simulink model "DWT"  (R2023a)
settings: Solver=ode45  StartTime=0.0  StopTime=4096+1024+100  RelTol=1e-3  EnableMultiTasking=on
PreLoadFcn:
  | xlrequire('imageData.mat'); xlrequire('PreLoadFcn');
PostLoadFcn:
  | open_system('DWT/Processor/Memory Controller','force'); pause(0.50); open_system('DWT');pause(0.50); close_system('DWT/Processor/Memory Controller');pause(0.50); close_system('DWT/Processor');
StopFcn:
  | xlrequire('StopFcn');
undefined symbols (not defined in the file): b1Init, b2Init
libraries: hdlBasic x212, dspindex x4, dspsnks4 x2, hdlUtilities x1, dspsrcs4 x1, vmcUtilities x1
(part 2 of 2)

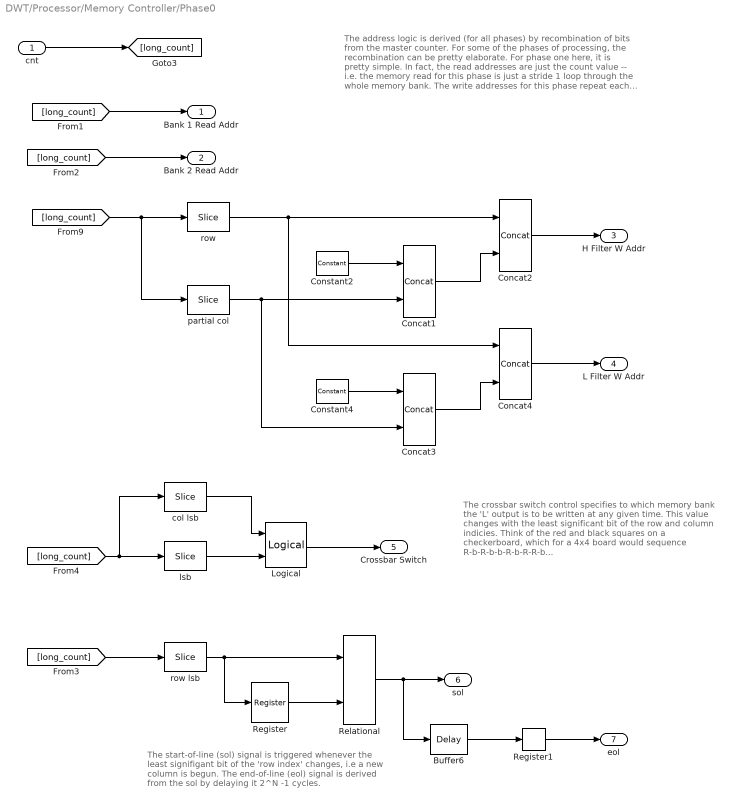
== system DWT/Processor/Memory Controller/Phase0 ==
  note: The address logic is derived (for all phases) by recombination
      | of bits from the master counter. For some of the phases of
      | processing, the recombination can be pretty elaborate.  For
      | phase one here, it is pretty simple.  In fact, the read addresses
      | are just the count value -- i.e. the memory read for this phase
      | is just a stride 1 loop through the whole memory bank.  The
      | write addresses for this phase repeat each address twice (data
      | is written to an address in one bank and then the same address
      | in the other bank for each filter).  The addresses increment by
      | one as each column is processed, and then jump to the next
      | column. A '1' is injected into the H address and a '0' into the 'L'
      | adress to write to the lower or upper half of memory, respectively.
  note: The crossbar switch control specifies to which memory
      | bank the 'L' output is to be written at any given time.
      | This value changes with the least significant bit of the
      | row and column indicies.  Think of the red and black
      | squares on a checkerboard, which for a 4x4 board would
      | sequence R-b-R-b-b-R-b-R-R-b...
  note: The start-of-line (sol) signal is triggered whenever the
      | least signifigant bit of the 'row index' changes, i.e a
      | new column is begun.  The end-of-line (eol) signal is
      | derived from the sol by delaying it 2^N -1 cycles.
  cnt : Inport
  Buffer6 : hdlBasic/Delay  rst=off  en=off  latency=power(2,N-1)-2  reg_retiming=off  XmcBlockStatus=1  maskContainerNames=group1  block_type=delay  block_config=sysgen:Delay_config
  Concat{1..4} (4 alike) : hdlBasic/Concat  num_inputs=2  XmcBlockStatus=1  maskContainerNames=group1  block_type=concat  block_config=sysgen:Concat_config
  Constant2 : hdlBasic/Constant  const=1  gui_display_data_type=Fixed-point  arith_type=Unsigned  n_bits=1  bin_pt=0  preci_type=Single  exp_width=8  frac_width=24  explicit_period=off  period=1  XmcBlockStatus=1  maskContainerNames=tabcontainer1  block_type=constant  block_config=sysgen:Constant_config
  Constant4 : hdlBasic/Constant  const=0  gui_display_data_type=Fixed-point  arith_type=Unsigned  n_bits=1  bin_pt=0  preci_type=Single  exp_width=8  frac_width=24  explicit_period=off  period=1  XmcBlockStatus=1  maskContainerNames=tabcontainer1  block_type=constant  block_config=sysgen:Constant_config
  Logical : hdlBasic/Logical  logical_function=XNOR  inputs=2  en=off  latency=0  precision=Full  arith_type=Unsigned  n_bits=8  bin_pt=2  align_bp=on  overflow=[]  quantization=[]  XmcBlockStatus=1  maskContainerNames=tabcontainer1  block_type=logical  block_config=sysgen:Logical_config
  Register : hdlBasic/Register  init=1  rst=off  en=off  XmcBlockStatus=1  maskContainerNames=tabcontainer1  block_type=register  block_config=sysgen:Register_config
  Register1 : hdlBasic/Register  init=0  rst=off  en=off  XmcBlockStatus=1  maskContainerNames=tabcontainer1  block_type=register  block_config=sysgen:Register_config
  Relational : hdlBasic/Relational  mode=a!=b  op_type=Bool  en=off  latency=0  XmcBlockStatus=1  maskContainerNames=tabcontainer1  block_type=relational  block_config=sysgen:Relational_config
  col lsb : hdlBasic/Slice  nbits=1  boolean_output=off  mode=Lower Bit Location + Width  bit1=0  base1=MSB of Input  bit0=M-1  base0=LSB of Input  XmcBlockStatus=1  maskContainerNames=group1  block_type=slice  block_config=sysgen:Slice_config
  lsb : hdlBasic/Slice  nbits=1  boolean_output=off  mode=Lower Bit Location + Width  bit1=0  base1=MSB of Input  bit0=0  base0=LSB of Input  XmcBlockStatus=1  maskContainerNames=group1  block_type=slice  block_config=sysgen:Slice_config
  partial col : hdlBasic/Slice  nbits=N-2  boolean_output=off  mode=Lower Bit Location + Width  bit1=0  base1=MSB of Input  bit0=1  base0=LSB of Input  XmcBlockStatus=1  maskContainerNames=group1  block_type=slice  block_config=sysgen:Slice_config
  row : hdlBasic/Slice  nbits=M  boolean_output=off  mode=Upper Bit Location + Width  bit1=0  base1=MSB of Input  bit0=N  base0=LSB of Input  XmcBlockStatus=1  maskContainerNames=group1  block_type=slice  block_config=sysgen:Slice_config
  row lsb : hdlBasic/Slice  nbits=1  boolean_output=off  mode=Lower Bit Location + Width  bit1=0  base1=MSB of Input  bit0=N-1  base0=LSB of Input  XmcBlockStatus=1  maskContainerNames=group1  block_type=slice  block_config=sysgen:Slice_config
  Bank 1 Read Addr : Outport  VectorParamsAs1DForOutWhenUnconnected=off
  Bank 2 Read Addr : Outport  Port=2  VectorParamsAs1DForOutWhenUnconnected=off
  H Filter W Addr : Outport  Port=3  VectorParamsAs1DForOutWhenUnconnected=off
  L Filter W Addr : Outport  Port=4  VectorParamsAs1DForOutWhenUnconnected=off
  Crossbar Switch : Outport  Port=5  VectorParamsAs1DForOutWhenUnconnected=off
  sol : Outport  Port=6  VectorParamsAs1DForOutWhenUnconnected=off
  eol : Outport  Port=7  VectorParamsAs1DForOutWhenUnconnected=off
  wires:
  [long_count] -> Bank 2 Read Addr/1
  [long_count] -> row lsb/1
  row lsb/1 -> Relational/1, Register/1
  Relational/1 -> sol/1, Buffer6/1
  Buffer6/1 -> Register1/1
  [long_count] -> lsb/1, col lsb/1
  Register/1 -> Relational/2
  [long_count] -> row/1, partial col/1
  row/1 -> Concat4/1, Concat2/1
  Constant2/1 -> Concat1/1
  Constant4/1 -> Concat3/1
  Concat3/1 -> Concat4/2
  partial col/1 -> Concat3/2, Concat1/2
  Concat1/1 -> Concat2/2
  [long_count] -> Bank 1 Read Addr/1
  Concat2/1 -> H Filter W Addr/1
  Concat4/1 -> L Filter W Addr/1
  Register1/1 -> eol/1
  cnt/1 -> [long_count]
  lsb/1 -> Logical/2
  col lsb/1 -> Logical/1
  Logical/1 -> Crossbar Switch/1

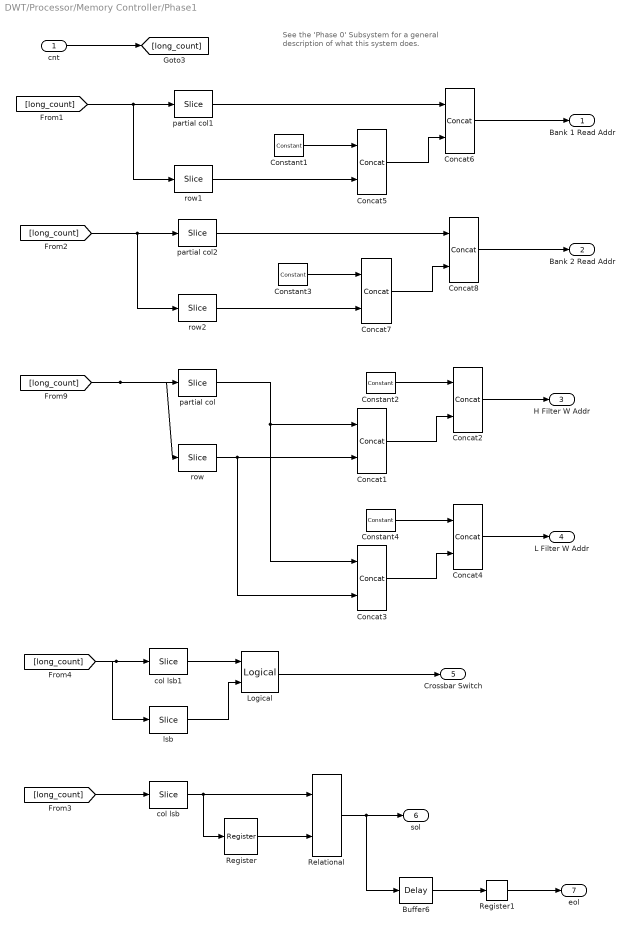
== system DWT/Processor/Memory Controller/Phase1 ==
  note: See the 'Phase 0' Subsystem for a general
      | description of what this system does.
  cnt : Inport
  Buffer6 : hdlBasic/Delay  rst=off  en=off  latency=power(2,N-1)-2  reg_retiming=off  XmcBlockStatus=1  maskContainerNames=group1  block_type=delay  block_config=sysgen:Delay_config
  Concat{1..8} (8 alike) : hdlBasic/Concat  num_inputs=2  XmcBlockStatus=1  maskContainerNames=group1  block_type=concat  block_config=sysgen:Concat_config
  Constant1 : hdlBasic/Constant  const=1  gui_display_data_type=Fixed-point  arith_type=Unsigned  n_bits=1  bin_pt=0  preci_type=Single  exp_width=8  frac_width=24  explicit_period=off  period=1  XmcBlockStatus=1  maskContainerNames=tabcontainer1  block_type=constant  block_config=sysgen:Constant_config
  Constant2 : hdlBasic/Constant  const=1  gui_display_data_type=Fixed-point  arith_type=Unsigned  n_bits=1  bin_pt=0  preci_type=Single  exp_width=8  frac_width=24  explicit_period=off  period=1  XmcBlockStatus=1  maskContainerNames=tabcontainer1  block_type=constant  block_config=sysgen:Constant_config
  Constant3 : hdlBasic/Constant  const=0  gui_display_data_type=Fixed-point  arith_type=Unsigned  n_bits=1  bin_pt=0  preci_type=Single  exp_width=8  frac_width=24  explicit_period=off  period=1  XmcBlockStatus=1  maskContainerNames=tabcontainer1  block_type=constant  block_config=sysgen:Constant_config
  Constant4 : hdlBasic/Constant  const=0  gui_display_data_type=Fixed-point  arith_type=Unsigned  n_bits=1  bin_pt=0  preci_type=Single  exp_width=8  frac_width=24  explicit_period=off  period=1  XmcBlockStatus=1  maskContainerNames=tabcontainer1  block_type=constant  block_config=sysgen:Constant_config
  Logical : hdlBasic/Logical  logical_function=XNOR  inputs=2  en=off  latency=0  precision=Full  arith_type=Unsigned  n_bits=8  bin_pt=2  align_bp=on  overflow=[]  quantization=[]  XmcBlockStatus=1  maskContainerNames=tabcontainer1  block_type=logical  block_config=sysgen:Logical_config
  Register : hdlBasic/Register  init=1  rst=off  en=off  XmcBlockStatus=1  maskContainerNames=tabcontainer1  block_type=register  block_config=sysgen:Register_config
  Register1 : hdlBasic/Register  init=0  rst=off  en=off  XmcBlockStatus=1  maskContainerNames=tabcontainer1  block_type=register  block_config=sysgen:Register_config
  Relational : hdlBasic/Relational  mode=a!=b  op_type=Bool  en=off  latency=0  XmcBlockStatus=1  maskContainerNames=tabcontainer1  block_type=relational  block_config=sysgen:Relational_config
  col lsb : hdlBasic/Slice  nbits=1  boolean_output=off  mode=Lower Bit Location + Width  bit1=0  base1=MSB of Input  bit0=M-1  base0=LSB of Input  XmcBlockStatus=1  maskContainerNames=group1  block_type=slice  block_config=sysgen:Slice_config
  col lsb1 : hdlBasic/Slice  nbits=1  boolean_output=off  mode=Lower Bit Location + Width  bit1=0  base1=MSB of Input  bit0=M-1  base0=LSB of Input  XmcBlockStatus=1  maskContainerNames=group1  block_type=slice  block_config=sysgen:Slice_config
  lsb : hdlBasic/Slice  nbits=1  boolean_output=off  mode=Lower Bit Location + Width  bit1=0  base1=MSB of Input  bit0=0  base0=LSB of Input  XmcBlockStatus=1  maskContainerNames=group1  block_type=slice  block_config=sysgen:Slice_config
  partial col : hdlBasic/Slice  nbits=N-1  boolean_output=off  mode=Lower Bit Location + Width  bit1=0  base1=MSB of Input  bit0=0  base0=LSB of Input  XmcBlockStatus=1  maskContainerNames=group1  block_type=slice  block_config=sysgen:Slice_config
  partial col1 : hdlBasic/Slice  nbits=N-1  boolean_output=off  mode=Lower Bit Location + Width  bit1=0  base1=MSB of Input  bit0=0  base0=LSB of Input  XmcBlockStatus=1  maskContainerNames=group1  block_type=slice  block_config=sysgen:Slice_config
  partial col2 : hdlBasic/Slice  nbits=N-1  boolean_output=off  mode=Lower Bit Location + Width  bit1=0  base1=MSB of Input  bit0=0  base0=LSB of Input  XmcBlockStatus=1  maskContainerNames=group1  block_type=slice  block_config=sysgen:Slice_config
  row : hdlBasic/Slice  nbits=M-1  boolean_output=off  mode=Upper Bit Location + Width  bit1=0  base1=MSB of Input  bit0=N  base0=LSB of Input  XmcBlockStatus=1  maskContainerNames=group1  block_type=slice  block_config=sysgen:Slice_config
  row1 : hdlBasic/Slice  nbits=M-1  boolean_output=off  mode=Upper Bit Location + Width  bit1=0  base1=MSB of Input  bit0=N  base0=LSB of Input  XmcBlockStatus=1  maskContainerNames=group1  block_type=slice  block_config=sysgen:Slice_config
  row2 : hdlBasic/Slice  nbits=M-1  boolean_output=off  mode=Upper Bit Location + Width  bit1=0  base1=MSB of Input  bit0=N  base0=LSB of Input  XmcBlockStatus=1  maskContainerNames=group1  block_type=slice  block_config=sysgen:Slice_config
  Bank 1 Read Addr : Outport  VectorParamsAs1DForOutWhenUnconnected=off
  Bank 2 Read Addr : Outport  Port=2  VectorParamsAs1DForOutWhenUnconnected=off
  H Filter W Addr : Outport  Port=3  VectorParamsAs1DForOutWhenUnconnected=off
  L Filter W Addr : Outport  Port=4  VectorParamsAs1DForOutWhenUnconnected=off
  Crossbar Switch : Outport  Port=5  VectorParamsAs1DForOutWhenUnconnected=off
  sol : Outport  Port=6  VectorParamsAs1DForOutWhenUnconnected=off
  eol : Outport  Port=7  VectorParamsAs1DForOutWhenUnconnected=off
  wires:
  cnt/1 -> [long_count]
  Register1/1 -> eol/1
  Concat4/1 -> L Filter W Addr/1
  Concat2/1 -> H Filter W Addr/1
  Concat1/1 -> Concat2/2
  Concat3/1 -> Concat4/2
  [long_count] -> partial col/1, row/1
  Register/1 -> Relational/2
  lsb/1 -> Logical/2
  [long_count] -> lsb/1, col lsb1/1
  Buffer6/1 -> Register1/1
  Relational/1 -> Buffer6/1, sol/1
  col lsb/1 -> Register/1, Relational/1
  [long_count] -> col lsb/1
  Concat5/1 -> Concat6/2
  partial col1/1 -> Concat6/1
  Concat6/1 -> Bank 1 Read Addr/1
  row1/1 -> Concat5/2
  [long_count] -> partial col1/1, row1/1
  Concat7/1 -> Concat8/2
  partial col2/1 -> Concat8/1
  Concat8/1 -> Bank 2 Read Addr/1
  row2/1 -> Concat7/2
  [long_count] -> partial col2/1, row2/1
  Constant2/1 -> Concat2/1
  Constant4/1 -> Concat4/1
  row/1 -> Concat1/2, Concat3/2
  Constant1/1 -> Concat5/1
  Constant3/1 -> Concat7/1
  col lsb1/1 -> Logical/1
  Logical/1 -> Crossbar Switch/1
  partial col/1 -> Concat1/1, Concat3/1

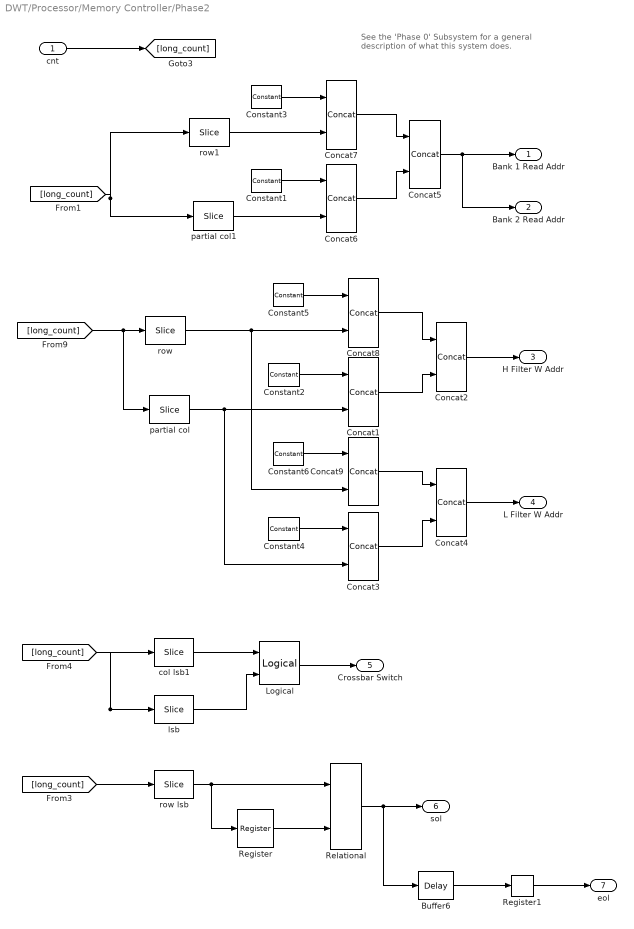
== system DWT/Processor/Memory Controller/Phase2 ==
  note: See the 'Phase 0' Subsystem for a general
      | description of what this system does.
  cnt : Inport
  Buffer6 : hdlBasic/Delay  rst=off  en=off  latency=power(2,N-1)-2  reg_retiming=off  XmcBlockStatus=1  maskContainerNames=group1  block_type=delay  block_config=sysgen:Delay_config
  Concat{1..9} (9 alike) : hdlBasic/Concat  num_inputs=2  XmcBlockStatus=1  maskContainerNames=group1  block_type=concat  block_config=sysgen:Concat_config
  Constant{1,3,5..6} (4 alike) : hdlBasic/Constant  const=0  gui_display_data_type=Fixed-point  arith_type=Unsigned  n_bits=1  bin_pt=0  preci_type=Single  exp_width=8  frac_width=24  explicit_period=off  period=1  XmcBlockStatus=1  maskContainerNames=tabcontainer1  block_type=constant  block_config=sysgen:Constant_config
  Constant2 : hdlBasic/Constant  const=1  gui_display_data_type=Fixed-point  arith_type=Unsigned  n_bits=2  bin_pt=0  preci_type=Single  exp_width=8  frac_width=24  explicit_period=off  period=1  XmcBlockStatus=1  maskContainerNames=tabcontainer1  block_type=constant  block_config=sysgen:Constant_config
  Constant4 : hdlBasic/Constant  const=0  gui_display_data_type=Fixed-point  arith_type=Unsigned  n_bits=2  bin_pt=0  preci_type=Single  exp_width=8  frac_width=24  explicit_period=off  period=1  XmcBlockStatus=1  maskContainerNames=tabcontainer1  block_type=constant  block_config=sysgen:Constant_config
  Logical : hdlBasic/Logical  logical_function=XNOR  inputs=2  en=off  latency=0  precision=Full  arith_type=Unsigned  n_bits=8  bin_pt=2  align_bp=on  overflow=[]  quantization=[]  XmcBlockStatus=1  maskContainerNames=tabcontainer1  block_type=logical  block_config=sysgen:Logical_config
  Register : hdlBasic/Register  init=1  rst=off  en=off  XmcBlockStatus=1  maskContainerNames=tabcontainer1  block_type=register  block_config=sysgen:Register_config
  Register1 : hdlBasic/Register  init=0  rst=off  en=off  XmcBlockStatus=1  maskContainerNames=tabcontainer1  block_type=register  block_config=sysgen:Register_config
  Relational : hdlBasic/Relational  mode=a!=b  op_type=Bool  en=off  latency=0  XmcBlockStatus=1  maskContainerNames=tabcontainer1  block_type=relational  block_config=sysgen:Relational_config
  col lsb1 : hdlBasic/Slice  nbits=1  boolean_output=off  mode=Lower Bit Location + Width  bit1=0  base1=MSB of Input  bit0=N-2  base0=LSB of Input  XmcBlockStatus=1  maskContainerNames=group1  block_type=slice  block_config=sysgen:Slice_config
  lsb : hdlBasic/Slice  nbits=1  boolean_output=off  mode=Lower Bit Location + Width  bit1=0  base1=MSB of Input  bit0=0  base0=LSB of Input  XmcBlockStatus=1  maskContainerNames=group1  block_type=slice  block_config=sysgen:Slice_config
  partial col : hdlBasic/Slice  nbits=N-3  boolean_output=off  mode=Lower Bit Location + Width  bit1=0  base1=MSB of Input  bit0=1  base0=LSB of Input  XmcBlockStatus=1  maskContainerNames=group1  block_type=slice  block_config=sysgen:Slice_config
  partial col1 : hdlBasic/Slice  nbits=N-2  boolean_output=off  mode=Lower Bit Location + Width  bit1=0  base1=MSB of Input  bit0=0  base0=LSB of Input  XmcBlockStatus=1  maskContainerNames=group1  block_type=slice  block_config=sysgen:Slice_config
  row : hdlBasic/Slice  nbits=M-1  boolean_output=off  mode=Upper Bit Location + Width  bit1=0  base1=MSB of Input  bit0=N  base0=LSB of Input  XmcBlockStatus=1  maskContainerNames=group1  block_type=slice  block_config=sysgen:Slice_config
  row lsb : hdlBasic/Slice  nbits=1  boolean_output=off  mode=Lower Bit Location + Width  bit1=0  base1=MSB of Input  bit0=N-2  base0=LSB of Input  XmcBlockStatus=1  maskContainerNames=group1  block_type=slice  block_config=sysgen:Slice_config
  row1 : hdlBasic/Slice  nbits=M-1  boolean_output=off  mode=Upper Bit Location + Width  bit1=0  base1=MSB of Input  bit0=N  base0=LSB of Input  XmcBlockStatus=1  maskContainerNames=group1  block_type=slice  block_config=sysgen:Slice_config
  Bank 1 Read Addr : Outport  VectorParamsAs1DForOutWhenUnconnected=off
  Bank 2 Read Addr : Outport  Port=2  VectorParamsAs1DForOutWhenUnconnected=off
  H Filter W Addr : Outport  Port=3  VectorParamsAs1DForOutWhenUnconnected=off
  L Filter W Addr : Outport  Port=4  VectorParamsAs1DForOutWhenUnconnected=off
  Crossbar Switch : Outport  Port=5  VectorParamsAs1DForOutWhenUnconnected=off
  sol : Outport  Port=6  VectorParamsAs1DForOutWhenUnconnected=off
  eol : Outport  Port=7  VectorParamsAs1DForOutWhenUnconnected=off
  wires:
  Logical/1 -> Crossbar Switch/1
  col lsb1/1 -> Logical/1
  lsb/1 -> Logical/2
  cnt/1 -> [long_count]
  Register1/1 -> eol/1
  Concat4/1 -> L Filter W Addr/1
  Concat2/1 -> H Filter W Addr/1
  Concat1/1 -> Concat2/2
  partial col/1 -> Concat1/2, Concat3/2
  Concat3/1 -> Concat4/2
  Constant4/1 -> Concat3/1
  Constant2/1 -> Concat1/1
  row/1 -> Concat8/2, Concat9/2
  [long_count] -> partial col/1, row/1
  Register/1 -> Relational/2
  [long_count] -> col lsb1/1, lsb/1
  Buffer6/1 -> Register1/1
  Relational/1 -> Buffer6/1, sol/1
  row lsb/1 -> Register/1, Relational/1
  [long_count] -> row lsb/1
  Concat5/1 -> Bank 1 Read Addr/1, Bank 2 Read Addr/1
  Constant1/1 -> Concat6/1
  partial col1/1 -> Concat6/2
  [long_count] -> partial col1/1, row1/1
  Concat6/1 -> Concat5/2
  row1/1 -> Concat7/2
  Constant3/1 -> Concat7/1
  Concat7/1 -> Concat5/1
  Constant5/1 -> Concat8/1
  Concat8/1 -> Concat2/1
  Constant6/1 -> Concat9/1
  Concat9/1 -> Concat4/1

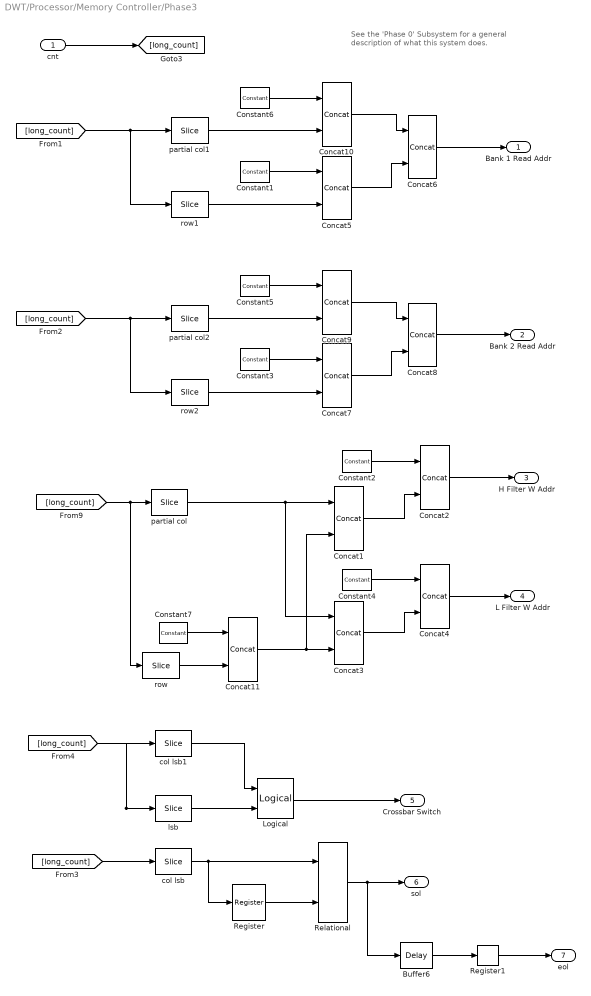
== system DWT/Processor/Memory Controller/Phase3 ==
  note: See the 'Phase 0' Subsystem for a general
      | description of what this system does.
  cnt : Inport
  Buffer6 : hdlBasic/Delay  rst=off  en=off  latency=power(2,N-1)-2  reg_retiming=off  XmcBlockStatus=1  maskContainerNames=group1  block_type=delay  block_config=sysgen:Delay_config
  Concat{1..11} (11 alike) : hdlBasic/Concat  num_inputs=2  XmcBlockStatus=1  maskContainerNames=group1  block_type=concat  block_config=sysgen:Concat_config
  Constant1 : hdlBasic/Constant  const=2  gui_display_data_type=Fixed-point  arith_type=Unsigned  n_bits=2  bin_pt=0  preci_type=Single  exp_width=8  frac_width=24  explicit_period=off  period=1  XmcBlockStatus=1  maskContainerNames=tabcontainer1  block_type=constant  block_config=sysgen:Constant_config
  Constant2 : hdlBasic/Constant  const=1  gui_display_data_type=Fixed-point  arith_type=Unsigned  n_bits=2  bin_pt=0  preci_type=Single  exp_width=8  frac_width=24  explicit_period=off  period=1  XmcBlockStatus=1  maskContainerNames=tabcontainer1  block_type=constant  block_config=sysgen:Constant_config
  Constant3 : hdlBasic/Constant  const=0  gui_display_data_type=Fixed-point  arith_type=Unsigned  n_bits=2  bin_pt=0  preci_type=Single  exp_width=8  frac_width=24  explicit_period=off  period=1  XmcBlockStatus=1  maskContainerNames=tabcontainer1  block_type=constant  block_config=sysgen:Constant_config
  Constant4 : hdlBasic/Constant  const=0  gui_display_data_type=Fixed-point  arith_type=Unsigned  n_bits=2  bin_pt=0  preci_type=Single  exp_width=8  frac_width=24  explicit_period=off  period=1  XmcBlockStatus=1  maskContainerNames=tabcontainer1  block_type=constant  block_config=sysgen:Constant_config
  Constant5 : hdlBasic/Constant  const=0  gui_display_data_type=Fixed-point  arith_type=Unsigned  n_bits=1  bin_pt=0  preci_type=Single  exp_width=8  frac_width=24  explicit_period=off  period=1  XmcBlockStatus=1  maskContainerNames=tabcontainer1  block_type=constant  block_config=sysgen:Constant_config
  Constant6 : hdlBasic/Constant  const=0  gui_display_data_type=Fixed-point  arith_type=Unsigned  n_bits=1  bin_pt=0  preci_type=Single  exp_width=8  frac_width=24  explicit_period=off  period=1  XmcBlockStatus=1  maskContainerNames=tabcontainer1  block_type=constant  block_config=sysgen:Constant_config
  Constant7 : hdlBasic/Constant  const=0  gui_display_data_type=Fixed-point  arith_type=Unsigned  n_bits=1  bin_pt=0  preci_type=Single  exp_width=8  frac_width=24  explicit_period=off  period=1  XmcBlockStatus=1  maskContainerNames=tabcontainer1  block_type=constant  block_config=sysgen:Constant_config
  Logical : hdlBasic/Logical  logical_function=XNOR  inputs=2  en=off  latency=0  precision=Full  arith_type=Unsigned  n_bits=8  bin_pt=2  align_bp=on  overflow=[]  quantization=[]  XmcBlockStatus=1  maskContainerNames=tabcontainer1  block_type=logical  block_config=sysgen:Logical_config
  Register : hdlBasic/Register  init=1  rst=off  en=off  XmcBlockStatus=1  maskContainerNames=tabcontainer1  block_type=register  block_config=sysgen:Register_config
  Register1 : hdlBasic/Register  init=0  rst=off  en=off  XmcBlockStatus=1  maskContainerNames=tabcontainer1  block_type=register  block_config=sysgen:Register_config
  Relational : hdlBasic/Relational  mode=a!=b  op_type=Bool  en=off  latency=0  XmcBlockStatus=1  maskContainerNames=tabcontainer1  block_type=relational  block_config=sysgen:Relational_config
  col lsb : hdlBasic/Slice  nbits=1  boolean_output=off  mode=Lower Bit Location + Width  bit1=0  base1=MSB of Input  bit0=M-2  base0=LSB of Input  XmcBlockStatus=1  maskContainerNames=group1  block_type=slice  block_config=sysgen:Slice_config
  col lsb1 : hdlBasic/Slice  nbits=1  boolean_output=off  mode=Lower Bit Location + Width  bit1=0  base1=MSB of Input  bit0=M-2  base0=LSB of Input  XmcBlockStatus=1  maskContainerNames=group1  block_type=slice  block_config=sysgen:Slice_config
  lsb : hdlBasic/Slice  nbits=1  boolean_output=off  mode=Lower Bit Location + Width  bit1=0  base1=MSB of Input  bit0=0  base0=LSB of Input  XmcBlockStatus=1  maskContainerNames=group1  block_type=slice  block_config=sysgen:Slice_config
  partial col : hdlBasic/Slice  nbits=N-2  boolean_output=off  mode=Lower Bit Location + Width  bit1=0  base1=MSB of Input  bit0=0  base0=LSB of Input  XmcBlockStatus=1  maskContainerNames=group1  block_type=slice  block_config=sysgen:Slice_config
  partial col1 : hdlBasic/Slice  nbits=N-2  boolean_output=off  mode=Lower Bit Location + Width  bit1=0  base1=MSB of Input  bit0=0  base0=LSB of Input  XmcBlockStatus=1  maskContainerNames=group1  block_type=slice  block_config=sysgen:Slice_config
  partial col2 : hdlBasic/Slice  nbits=N-2  boolean_output=off  mode=Lower Bit Location + Width  bit1=0  base1=MSB of Input  bit0=0  base0=LSB of Input  XmcBlockStatus=1  maskContainerNames=group1  block_type=slice  block_config=sysgen:Slice_config
  row : hdlBasic/Slice  nbits=M-2  boolean_output=off  mode=Upper Bit Location + Width  bit1=0  base1=MSB of Input  bit0=N  base0=LSB of Input  XmcBlockStatus=1  maskContainerNames=group1  block_type=slice  block_config=sysgen:Slice_config
  row1 : hdlBasic/Slice  nbits=M-2  boolean_output=off  mode=Upper Bit Location + Width  bit1=0  base1=MSB of Input  bit0=N  base0=LSB of Input  XmcBlockStatus=1  maskContainerNames=group1  block_type=slice  block_config=sysgen:Slice_config
  row2 : hdlBasic/Slice  nbits=M-2  boolean_output=off  mode=Upper Bit Location + Width  bit1=0  base1=MSB of Input  bit0=N  base0=LSB of Input  XmcBlockStatus=1  maskContainerNames=group1  block_type=slice  block_config=sysgen:Slice_config
  Bank 1 Read Addr : Outport  VectorParamsAs1DForOutWhenUnconnected=off
  Bank 2 Read Addr : Outport  Port=2  VectorParamsAs1DForOutWhenUnconnected=off
  H Filter W Addr : Outport  Port=3  VectorParamsAs1DForOutWhenUnconnected=off
  L Filter W Addr : Outport  Port=4  VectorParamsAs1DForOutWhenUnconnected=off
  Crossbar Switch : Outport  Port=5  VectorParamsAs1DForOutWhenUnconnected=off
  sol : Outport  Port=6  VectorParamsAs1DForOutWhenUnconnected=off
  eol : Outport  Port=7  VectorParamsAs1DForOutWhenUnconnected=off
  wires:
  Logical/1 -> Crossbar Switch/1
  col lsb1/1 -> Logical/1
  Constant3/1 -> Concat7/1
  Constant1/1 -> Concat5/1
  partial col/1 -> Concat3/1, Concat1/1
  Constant4/1 -> Concat4/1
  Constant2/1 -> Concat2/1
  [long_count] -> row2/1, partial col2/1
  row2/1 -> Concat7/2
  Concat8/1 -> Bank 2 Read Addr/1
  Concat7/1 -> Concat8/2
  [long_count] -> row1/1, partial col1/1
  row1/1 -> Concat5/2
  Concat6/1 -> Bank 1 Read Addr/1
  Concat5/1 -> Concat6/2
  [long_count] -> col lsb/1
  col lsb/1 -> Relational/1, Register/1
  Relational/1 -> sol/1, Buffer6/1
  Buffer6/1 -> Register1/1
  [long_count] -> col lsb1/1, lsb/1
  lsb/1 -> Logical/2
  Register/1 -> Relational/2
  [long_count] -> row/1, partial col/1
  Concat3/1 -> Concat4/2
  Concat1/1 -> Concat2/2
  Concat2/1 -> H Filter W Addr/1
  Concat4/1 -> L Filter W Addr/1
  Register1/1 -> eol/1
  cnt/1 -> [long_count]
  Constant5/1 -> Concat9/1
  partial col2/1 -> Concat9/2
  Concat9/1 -> Concat8/1
  Constant6/1 -> Concat10/1
  partial col1/1 -> Concat10/2
  Concat10/1 -> Concat6/1
  Constant7/1 -> Concat11/1
  row/1 -> Concat11/2
  Concat11/1 -> Concat3/2, Concat1/2

== system DWT/Processor/Memory Controller/S-R FF ==
  note: 1-bit register used as Set-Reset Flip Flop.
  s : Inport
  r : Inport  Port=2
  Register2 : hdlBasic/Register  init=0  rst=on  en=on  XmcBlockStatus=1  maskContainerNames=tabcontainer1  block_type=register  block_config=sysgen:Register_config
  q : Outport  VectorParamsAs1DForOutWhenUnconnected=off
  wires:
  s/1 -> Register2/1, Register2/3
  r/1 -> Register2/2
  Register2/1 -> q/1

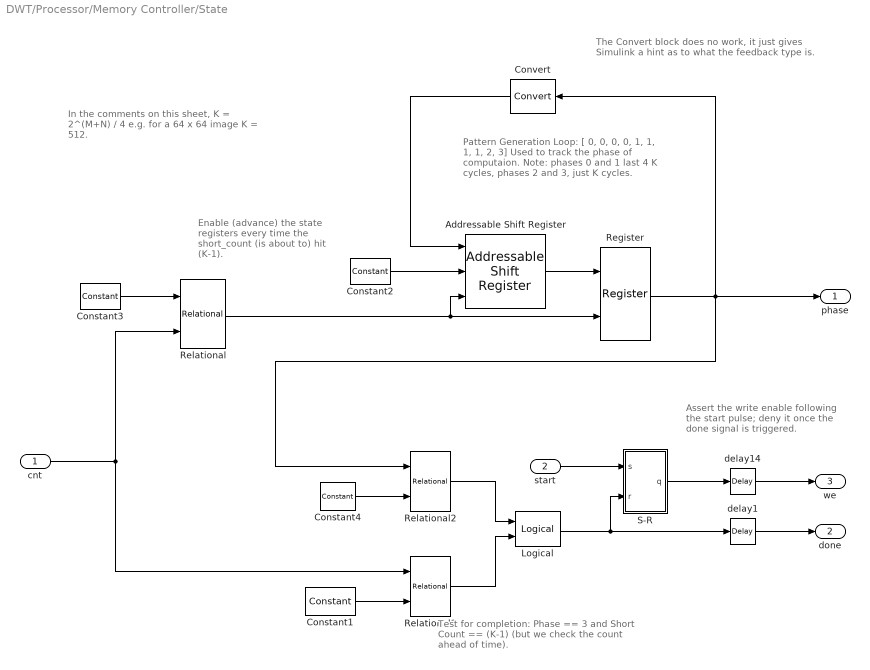
== system DWT/Processor/Memory Controller/State ==
  note: Pattern Generation Loop:
      | [ 0, 0, 0, 0, 1, 1, 1, 1, 2, 3]
      | Used to track the phase of computaion.
      | Note: phases 0 and 1 last 4 K cycles,
      | phases 2 and 3, just K cycles.
  note: Test for completion:
      | Phase == 3  and
      | Short Count == (K-1)
      | (but we check the count ahead of time).
  note: Enable (advance) the
      | state registers every time
      | the short_count (is about to)
      | hit  (K-1).
  note: Assert the write enable following
      | the start pulse;  deny it once the
      | done signal is triggered.
  note: In the comments on this sheet,
      |  K = 2^(M+N) / 4
      | e.g. for a 64 x 64 image K = 512.
  note: The Convert block does no work, it  just gives
      | Simulink a hint as to what the feedback type is.
  cnt : Inport
  start : Inport  Port=2
  Addressable Shift Register : hdlBasic/Addressable Shift Register  infer_latency=on  depth=2  initVector=[3 2 1 1 1 1 0 0 0]  en=on  use_behavioral_HDL=off  Optimization=Resource  use_rpm=off  XmcBlockStatus=1  maskContainerNames=group1  block_type=addrsr  block_config=sysgen:Addrsr_config
  Constant1 : hdlBasic/Constant  const=power(2,M+N-2) - 4  gui_display_data_type=Fixed-point  arith_type=Unsigned  n_bits=M+N-3  bin_pt=0  preci_type=Single  exp_width=8  frac_width=24  explicit_period=off  period=1  XmcBlockStatus=1  maskContainerNames=tabcontainer1  block_type=constant  block_config=sysgen:Constant_config
  Constant2 : hdlBasic/Constant  const=8  gui_display_data_type=Fixed-point  arith_type=Unsigned  n_bits=4  bin_pt=0  preci_type=Single  exp_width=8  frac_width=24  explicit_period=off  period=1  XmcBlockStatus=1  maskContainerNames=tabcontainer1  block_type=constant  block_config=sysgen:Constant_config
  Constant3 : hdlBasic/Constant  const=power(2,M+N-2) - 2  gui_display_data_type=Fixed-point  arith_type=Unsigned  n_bits=M+N-3  bin_pt=0  preci_type=Single  exp_width=8  frac_width=24  explicit_period=off  period=1  XmcBlockStatus=1  maskContainerNames=tabcontainer1  block_type=constant  block_config=sysgen:Constant_config
  Constant4 : hdlBasic/Constant  const=3  gui_display_data_type=Fixed-point  arith_type=Unsigned  n_bits=2  bin_pt=0  preci_type=Single  exp_width=8  frac_width=24  explicit_period=off  period=1  XmcBlockStatus=1  maskContainerNames=tabcontainer1  block_type=constant  block_config=sysgen:Constant_config
  Convert : hdlBasic/Convert  gui_display_data_type=Fixed-point  arith_type=Unsigned  n_bits=2  bin_pt=0  float_type=Single  exp_bits=8  fraction_bits=24  quantization=Truncate  overflow=Wrap  en=off  latency=0  pipeline=off  XmcBlockStatus=1  maskContainerNames=group2  block_type=convert  block_config=sysgen:Convert_config  block_width=595  block_height=885
  Logical : hdlBasic/Logical  logical_function=AND  inputs=2  en=off  latency=0  precision=Full  arith_type=Unsigned  n_bits=8  bin_pt=2  align_bp=on  overflow=[]  quantization=[]  XmcBlockStatus=1  maskContainerNames=tabcontainer1  block_type=logical  block_config=sysgen:Logical_config
  Register : hdlBasic/Register  init=0  rst=off  en=on  XmcBlockStatus=1  maskContainerNames=tabcontainer1  block_type=register  block_config=sysgen:Register_config
  Relational : hdlBasic/Relational  mode=a=b  op_type=Bool  en=off  latency=1  XmcBlockStatus=1  maskContainerNames=tabcontainer1  block_type=relational  block_config=sysgen:Relational_config
  Relational1 : hdlBasic/Relational  mode=a=b  op_type=Bool  en=off  latency=2  XmcBlockStatus=1  maskContainerNames=tabcontainer1  block_type=relational  block_config=sysgen:Relational_config
  Relational2 : hdlBasic/Relational  mode=a=b  op_type=Bool  en=off  latency=2  XmcBlockStatus=1  maskContainerNames=tabcontainer1  block_type=relational  block_config=sysgen:Relational_config
  S-R : Subsystem
  delay1 : hdlBasic/Delay  rst=off  en=off  latency=2  reg_retiming=off  XmcBlockStatus=1  maskContainerNames=group1  block_type=delay  block_config=sysgen:Delay_config
  delay14 : hdlBasic/Delay  rst=off  en=off  latency=1  reg_retiming=off  XmcBlockStatus=1  maskContainerNames=group1  block_type=delay  block_config=sysgen:Delay_config
  phase : Outport  VectorParamsAs1DForOutWhenUnconnected=off
  done : Outport  Port=2  VectorParamsAs1DForOutWhenUnconnected=off
  we : Outport  Port=3  VectorParamsAs1DForOutWhenUnconnected=off
  wires:
  Relational/1 -> Addressable Shift Register/3, Register/2
  Register/1 -> phase/1, Convert/1, Relational2/1
  S-R/1(q) -> delay14/1
  start/1 -> S-R/1(s)
  Constant4/1 -> Relational2/2
  Logical/1 -> S-R/2(r), delay1/1
  delay14/1 -> we/1
  Convert/1 -> Addressable Shift Register/1
  delay1/1 -> done/1
  Constant3/1 -> Relational/1
  cnt/1 -> Relational/2, Relational1/1
  Relational2/1 -> Logical/1
  Relational1/1 -> Logical/2
  Constant1/1 -> Relational1/2
  Constant2/1 -> Addressable Shift Register/2
  Addressable Shift Register/1 -> Register/1

== system DWT/Processor/Memory Controller/State/S-R ==
  note: 1-bit register used as Set-Reset Flip Flop.
  s : Inport
  r : Inport  Port=2
  Register2 : hdlBasic/Register  init=0  rst=on  en=on  XmcBlockStatus=1  maskContainerNames=tabcontainer1  block_type=register  block_config=sysgen:Register_config
  q : Outport  VectorParamsAs1DForOutWhenUnconnected=off
  wires:
  s/1 -> Register2/1, Register2/3
  r/1 -> Register2/2
  Register2/1 -> q/1
